simulink model "MPCquadprog"  (R2023a)
settings: Solver=ode4  StartTime=0.0  StopTime=tsim  FixedStep=baseRate  RelTol=1e-6  AbsTol=1e-6
values from neighbouring files (symbols this model uses):
  ALGORITHM = 5    [Run_Initializer.m]
  con0 = [n*N, 2*N, N, N, N]    [Run_Initializer.m]
  Gamma1_el = 0.12    [Run_Initializer.m]
  Gamma1_sh = 0.005    [Run_Initializer.m]
  Gamma1_wr = 0.025    [Run_Initializer.m]
  Gamma2_el = 5    [Run_Initializer.m]
  Gamma2_sh = 5    [Run_Initializer.m]
  Gamma2_wr = 5    [Run_Initializer.m]
  Gamma3_el = 10    [Run_Initializer.m]
  Gamma3_sh = 40    [Run_Initializer.m]
  Gamma3_wr = 40    [Run_Initializer.m]
  Gamma4_el = 0.039    [Run_Initializer.m]
  Gamma4_sh = 0.015    [Run_Initializer.m]
  Gamma4_wr = 0.029    [Run_Initializer.m]
  Gamma5_el = 800    [Run_Initializer.m]
  Gamma5_sh = 800    [Run_Initializer.m]
  Gamma5_wr = 800    [Run_Initializer.m]
  Gamma6_el = 0.000001    (= 1e-06)    [Run_Initializer.m]
  Gamma6_sh = 0.005    [Run_Initializer.m]
  Gamma6_wr = 0.02    [Run_Initializer.m]
  init_states_BLACK = [ct;thetat0].'    [Run_Initializer.m]
  init_states_BLUE = [pobj1;0].'    [Run_Initializer.m]
  init_states_RED = xi(1:3).'    [Run_Initializer.m]
  Kd_elarm = 0.8    [Run_Initializer.m]
  Kd_sharm = 1.0    (= 1)    [Run_Initializer.m]
  Kd_wrarm = 0.6    [Run_Initializer.m]
  Kp_elarm = 1.2    [Run_Initializer.m]
  Kp_sharm = 1.5    [Run_Initializer.m]
  Kp_wrarm = 2    [Run_Initializer.m]
  maxiterations = 10    [Run_Initializer.m]
  N = 15    [Run_Initializer.m]    (also in theConstraintLimits4.m)
  Td = 2    [Run_Initializer.m]
  thetat_dot = 2.5 * d2r    (= 0.0436332312999)    [Run_Initializer.m]
  tol = 0.00015    [Run_Initializer.m]
  Tz_lim_elarm = .1    (= 0.1)    [Run_Initializer.m]
  Tz_lim_sharm = .1    (= 0.1)    [Run_Initializer.m]
  Tz_lim_wrarm = .1    (= 0.1)    [Run_Initializer.m]
  vobj1 = [0.00;0.00]    [Run_Initializer.m]
  vtar = [-0.005;0.005]    [Run_Initializer.m]
undefined symbols (not defined in the file or in its folder): a1, a2, a3, Ad, b0, b1, b2, b3, baseRate, cdockdeltax, cdockoa, Cmat, DiscIntNeverNeededParam, drop_states_ARM, drop_states_BLACK, drop_states_BLUE, drop_states_RED, ecoa, F_Black_X_nominal, F_Black_Y_nominal, F_Blue_X_nominal, F_Blue_Y_nominal, F_red_X_nominal, F_red_Y_nominal, F_thrusters_BLACK, F_thrusters_BLUE, F_thrusters_RED, Fmat, gamma, H, IBLACK, IBLUE, IDIST, IEE, IPROX, IRED, Kd_tb, Kd_tblue, Kd_tr, Kd_xb, Kd_xblue, Kd_xr, Kd_yb, Kd_yblue, Kd_yr, KOZ_actual, Kp_tb, Kp_tblue, Kp_tr, Kp_xb, Kp_xblue, Kp_xr, Kp_yb, Kp_yblue, Kp_yr, mBLACK, mBLUE, mDIST, mEE, mPROX ... (+32)
libraries: nvidiaSharedBlocks x8, simulink x8, dspsigops x6, dspstat3 x5, MainLibrary x4
(part 10 of 10)

== matlab function MPCquadprog/Phase #3: Experiment/Change RED Behavior/Sub-Phase #4/Subsystem/MATLAB Function ==
  data: x input; x output
function x = fcn(x)
    if x > pi
        x  = x - 2*pi;
    elseif x <= -pi
        x = x + 2*pi;
    end

== matlab function MPCquadprog/Thruster Control Code/Change RED Behavior/Calculate Thruster ON//OFF/MATLAB Function3 ==
  data: H output; thruster_dist2CG_RED parameter; F_thrusters_RED parameter
function H = MakeH(thruster_dist2CG_RED,F_thrusters_RED)

Vec1 = [ -1
         -1
          0 
          0
          1
          1
          0
          0 ];
      
Vec2 = [  0
          0
          1
          1
          0
          0
         -1
         -1 ];
     
Vec3 = thruster_dist2CG_RED./1000;

Mat1 = [Vec1, Vec2, Vec3]';

Mat2 = diag((F_thrusters_RED./2));

H    = Mat1*Mat2;

end

== matlab function MPCquadprog/Thruster Control Code/Change RED Behavior/Calculate Thruster ON//OFF/MATLAB Function4 ==
  data: H output; thruster_dist2CG_RED parameter; F_red_X_nominal parameter; theta_1 input; theta_2 input; theta_3 input; mRED parameter; thrust_decay_factor input; F_red_Y_nominal parameter; mPROX parameter; mDIST parameter; mEE parameter; Phi parameter; b0 parameter; a1 parameter; b1 parameter; a2 parameter; b2 parameter; a3 parameter; b3 parameter
function H   = MakeH(thruster_dist2CG_RED,F_red_X_nominal, theta_1, theta_2, theta_3, mRED, thrust_decay_factor, F_red_Y_nominal, mPROX, mDIST, mEE, Phi, b0, a1, b1, a2, b2, a3, b3)
    
    link1_com_x = b0*cos(Phi) + a1*cos(pi/2 + theta_1);
    link1_com_y = b0*sin(Phi) + a1*sin(pi/2 + theta_1);
    
    link2_com_x = link1_com_x + b1*cos(pi/2 + theta_1) + a2*cos(pi/2 + theta_1 + theta_2);
    link2_com_y = link1_com_y + b1*sin(pi/2 + theta_1) + a2*sin(pi/2 + theta_1 + theta_2);
    
    link3_com_x = link2_com_x + b2*cos(pi/2 + theta_1 + theta_2) + a3*cos(pi/2 + theta_1 + theta_2 + theta_3);
    link3_com_y = link2_com_y + b2*sin(pi/2 + theta_1 + theta_2) + a3*sin(pi/2 + theta_1 + theta_2 + theta_3);
    
    delta_com_due_to_arm_x = (mPROX*link1_com_x + mDIST*link2_com_x + mEE*link3_com_x)/(mRED + mPROX + mDIST + mEE)*1000; % [mm]
    delta_com_due_to_arm_y = (mPROX*link1_com_y + mDIST*link2_com_y + mEE*link3_com_y)/(mRED + mPROX + mDIST + mEE)*1000; % [mm]
    
    adjusted_thruster_dist2CG_RED = [thruster_dist2CG_RED(1)-delta_com_due_to_arm_y;
                                     thruster_dist2CG_RED(2)-delta_com_due_to_arm_y;
                                     thruster_dist2CG_RED(3)-delta_com_due_to_arm_x;
                                     thruster_dist2CG_RED(4)-delta_com_due_to_arm_x;
                                     thruster_dist2CG_RED(5)+delta_com_due_to_arm_y;
                                     thruster_dist2CG_RED(6)+delta_com_due_to_arm_y;
                                     thruster_dist2CG_RED(7)+delta_com_due_to_arm_x;
                                     thruster_dist2CG_RED(8)+delta_com_due_to_arm_x];
                                     
    
    
    Vec1 = [ -1
             -1
              0 
              0
              1
              1
              0
              0 ];
          
    Vec2 = [  0
              0
              1
              1
              0
              0
             -1
             -1 ];
         
    Vec3 = adjusted_thruster_dist2CG_RED./1000;
    
    Mat1 = [Vec1, Vec2, Vec3]';
    
    F_thrusters_RED = [F_red_X_nominal*thrust_decay_factor; F_red_X_nominal*thrust_decay_factor; F_red_Y_nominal*thrust_decay_factor; F_red_Y_nominal*thrust_decay_factor; F_red_X_nominal*thrust_decay_factor; F_red_X_nominal*thrust_decay_factor; F_red_Y_nominal*thrust_decay_factor; F_red_Y_nominal*thrust_decay_factor];
    
    Mat2 = diag((F_thrusters_RED));
    
    H    = Mat1*Mat2;

end

== matlab function MPCquadprog/Thruster Control Code/Change RED Behavior/Calculate Thruster ON//OFF/MATLAB Function5 ==
  data: thrust_decay_factor output; PWMs input; thruster_count_threshold parameter; count output
function [thrust_decay_factor, count]  = check_thrust_decay(PWMs,thruster_count_threshold)

% normalize PWMs
if max(PWMs) > 1
    PWMs = PWMs/max(PWMs);
end

count = sum(PWMs > thruster_count_threshold);

positives_only = max(PWMs,0);
sum_of_duty_cycles = sum(positives_only);

average_duty_cycle_per_thruster = sum_of_duty_cycles/count;

% Look up the thrust decay for this average duty cycle
if (average_duty_cycle_per_thruster < 0.3) || (count == 0)
    thrust_decay_factor = 1;
else
    thrust_decay_factor = max(0.6 - 2*average_duty_cycle_per_thruster + 1, 0.5);   
end

== matlab function MPCquadprog/Thruster Control Code/Change RED Behavior/Calculate Thruster ON//OFF/MATLAB Function6 ==
  data: H output; thruster_dist2CG_RED parameter; F_red_X_nominal parameter; theta_1 input; theta_2 input; theta_3 input; mRED parameter; thrust_decay_factor input; F_red_Y_nominal parameter; mPROX parameter; mDIST parameter; mEE parameter; Phi parameter; b0 parameter; a1 parameter; b1 parameter; a2 parameter; b2 parameter; a3 parameter; b3 parameter
function H   = MakeHWithArmAndDecay(thruster_dist2CG_RED,F_red_X_nominal, theta_1, theta_2, theta_3,  mRED, thrust_decay_factor, F_red_Y_nominal, mPROX, mDIST, mEE, Phi, b0, a1, b1, a2, b2, a3, b3)
    
    link1_com_x = b0*cos(Phi) + a1*cos(pi/2 + theta_1);
    link1_com_y = b0*sin(Phi) + a1*sin(pi/2 + theta_1);
    
    link2_com_x = link1_com_x + b1*cos(pi/2 + theta_1) + a2*cos(pi/2 + theta_1 + theta_2);
    link2_com_y = link1_com_y + b1*sin(pi/2 + theta_1) + a2*sin(pi/2 + theta_1 + theta_2);
    
    link3_com_x = link2_com_x + b2*cos(pi/2 + theta_1 + theta_2) + a3*cos(pi/2 + theta_1 + theta_2 + theta_3);
    link3_com_y = link2_com_y + b2*sin(pi/2 + theta_1 + theta_2) + a3*sin(pi/2 + theta_1 + theta_2 + theta_3);
    
    delta_com_due_to_arm_x = (mPROX*link1_com_x + mDIST*link2_com_x + mEE*link3_com_x)/(mRED + mPROX + mDIST + mEE)*1000; % [mm]
    delta_com_due_to_arm_y = (mPROX*link1_com_y + mDIST*link2_com_y + mEE*link3_com_y)/(mRED + mPROX + mDIST + mEE)*1000; % [mm]
    
    adjusted_thruster_dist2CG_RED = [thruster_dist2CG_RED(1)-delta_com_due_to_arm_y;
                                     thruster_dist2CG_RED(2)-delta_com_due_to_arm_y;
                                     thruster_dist2CG_RED(3)-delta_com_due_to_arm_x;
                                     thruster_dist2CG_RED(4)-delta_com_due_to_arm_x;
                                     thruster_dist2CG_RED(5)+delta_com_due_to_arm_y;
                                     thruster_dist2CG_RED(6)+delta_com_due_to_arm_y;
                                     thruster_dist2CG_RED(7)+delta_com_due_to_arm_x;
                                     thruster_dist2CG_RED(8)+delta_com_due_to_arm_x];
                                 
    
    
    Vec1 = [ -1
             -1
              0 
              0
              1
              1
              0
              0 ];
          
    Vec2 = [  0
              0
              1
              1
              0
              0
             -1
             -1 ];
         
    Vec3 = adjusted_thruster_dist2CG_RED./1000;
    
    Mat1 = [Vec1, Vec2, Vec3]';
    
    F_thrusters_RED = [F_red_X_nominal*thrust_decay_factor; F_red_X_nominal*thrust_decay_factor; F_red_Y_nominal*thrust_decay_factor; F_red_Y_nominal*thrust_decay_factor; F_red_X_nominal*thrust_decay_factor; F_red_X_nominal*thrust_decay_factor; F_red_Y_nominal*thrust_decay_factor; F_red_Y_nominal*thrust_decay_factor];
    
    Mat2 = diag((F_thrusters_RED./2));
    
    H    = Mat1*Mat2;

end

== matlab function MPCquadprog/Phase #3: Experiment/Change RED Behavior/Sub-Phase #4/Subsystem/MATLAB Function2 ==
  data: x input; x output
function x = fcn(x)
    if x > pi
        x  = x - 2*pi;
    elseif x <= -pi
        x = x + 2*pi;
    end

== matlab function MPCquadprog/Phase #3: Experiment/Change BLACK Behavior/Sub-Phase #3 /Hough Control/MATLAB Function4 ==
  data: Oy input; e_out output; e_in input
function e_out = fcn(Oy, e_in)

a = sign(Oy'*e_in);
e_out = -a*norm(e_in);

== matlab function MPCquadprog/Phase #3: Experiment/Change BLACK Behavior/Sub-Phase #3 /Hough Control/MATLAB Function2 ==
  data: Oy output; z input; Ox output
function [Oy, Ox]   = C3( z )
%C3 gives the rotation matrix about the z-axis for an angle 'z'
%   z - the angle about the z-axis which you rotate
%   A - the rotation matrix

Ox = [cos(z) sin(z); -sin(z) cos(z)]*[1;0];
Oy = [cos(z) sin(z); -sin(z) cos(z)]*[0;1];
end

== matlab function MPCquadprog/Phase #3: Experiment/Change BLACK Behavior/Sub-Phase #3 /Hough Control/MATLAB Function3 ==
  data: z input; Ox output
function Ox    = C3( z )
%C3 gives the rotation matrix about the z-axis for an angle 'z'
%   z - the angle about the z-axis which you rotate
%   A - the rotation matrix

Ox = [cos(z) sin(z); -sin(z) cos(z)]*[1;0];
end

== matlab function MPCquadprog/Phase #3: Experiment/Change BLACK Behavior/Sub-Phase #1/Hough Control/MATLAB Function4 ==
  data: Oy input; e_out output; e_in input
function e_out = fcn(Oy, e_in)

a = sign(Oy'*e_in);
e_out = -a*norm(e_in);

== matlab function MPCquadprog/PhaseSpace Camera Code/Use Hardware to Obtain States/MATLAB Function ==
  data: StartClock output; RedReceiving input; BlackReceiving input; BlueReceiving input; platformSelection parameter
function StartClock = CheckForSync(RedReceiving, BlackReceiving, BlueReceiving, platformSelection)
        
    StartClock = 0;
    
    if (platformSelection == 1)
        
        if RedReceiving == 1

            StartClock = 1;

        else

            StartClock = 0;

        end
        
    elseif (platformSelection == 2)
        
        if BlackReceiving == 1

            StartClock = 1;

        else

            StartClock = 0;

        end  
        
    elseif (platformSelection == 3)
        
        if RedReceiving == 1 && BlackReceiving == 1

            StartClock = 1;

        else

            StartClock = 0;

        end    
        
    elseif (platformSelection == 4)
        
        if RedReceiving == 1 && BlackReceiving == 1

            StartClock = 1;

        else

            StartClock = 0;

        end
        
    elseif (platformSelection == 5)
        
        if RedReceiving == 1

            StartClock = 1;

        else

            StartClock = 0;

        end
        
    elseif (platformSelection == 6)
        
        if BlueReceiving == 1

            StartClock = 1;

        else

            StartClock = 0;

        end
        
    elseif (platformSelection == 7)
        
        if RedReceiving == 1 && BlueReceiving == 1

            StartClock = 1;

        else

            StartClock = 0;

        end
        
    elseif (platformSelection == 8)
        
        if RedReceiving == 1 && BlackReceiving == 1 && BlueReceiving == 1

            StartClock = 1;

        else

            StartClock = 0;

        end
        
    elseif (platformSelection == 9)
        
        if BlackReceiving == 1 && BlueReceiving == 1

            StartClock = 1;

        else

            StartClock = 0;

        end
                           
    elseif (platformSelection == 10)
        
        if RedReceiving == 1 && BlueReceiving == 1

            StartClock = 1;

        else

            StartClock = 0;

        end
        
    elseif (platformSelection == 11)
        
        if RedReceiving == 1 && BlackReceiving == 1 && BlueReceiving == 1

            StartClock = 1;

        else

            StartClock = 0;

        end
        
    end



end

== matlab function MPCquadprog/Thruster Control Code/Change BLUE Behavior/Calculate Thruster ON//OFF/MATLAB Function6 ==
  data: thrust_decay_factor output; PWMs input; thruster_count_threshold parameter; count output
function [thrust_decay_factor, count]  = check_thrust_decay(PWMs,thruster_count_threshold)

% normalize PWMs
if max(PWMs) > 1
    PWMs = PWMs/max(PWMs);
end

count = sum(PWMs > thruster_count_threshold);

positives_only = max(PWMs,0);
sum_of_duty_cycles = sum(positives_only);

average_duty_cycle_per_thruster = sum_of_duty_cycles/count;

% Look up the thrust decay for this average duty cycle
if (average_duty_cycle_per_thruster < 0.3) || (count == 0)
    thrust_decay_factor = 1;
else
    thrust_decay_factor = max(0.6 - 2*average_duty_cycle_per_thruster + 1, 0.5);   
end

== matlab function MPCquadprog/Thruster Control Code/Change BLUE Behavior/Calculate Thruster ON//OFF/MATLAB Function7 ==
  data: H output; thruster_dist2CG_BLUE parameter; F_Blue_X_nominal parameter; thrust_decay_factor input; F_Blue_Y_nominal parameter
function H   = MakeHWithDecay(thruster_dist2CG_BLUE,F_Blue_X_nominal, thrust_decay_factor, F_Blue_Y_nominal)


adjusted_thruster_dist2CG_BLUE = [thruster_dist2CG_BLUE(1);
                                 thruster_dist2CG_BLUE(2);
                                 thruster_dist2CG_BLUE(3);
                                 thruster_dist2CG_BLUE(4);
                                 thruster_dist2CG_BLUE(5);
                                 thruster_dist2CG_BLUE(6);
                                 thruster_dist2CG_BLUE(7);
                                 thruster_dist2CG_BLUE(8)];
                                 


Vec1 = [ -1
         -1
          0 
          0
          1
          1
          0
          0 ];
      
Vec2 = [  0
          0
          1
          1
          0
          0
         -1
         -1 ];
     
Vec3 = adjusted_thruster_dist2CG_BLUE./1000;

Mat1 = [Vec1, Vec2, Vec3]';

F_thrusters_BLUE = [F_Blue_X_nominal*thrust_decay_factor; F_Blue_X_nominal*thrust_decay_factor; F_Blue_Y_nominal*thrust_decay_factor; F_Blue_Y_nominal*thrust_decay_factor; F_Blue_X_nominal*thrust_decay_factor; F_Blue_X_nominal*thrust_decay_factor; F_Blue_Y_nominal*thrust_decay_factor; F_Blue_Y_nominal*thrust_decay_factor];

Mat2 = diag((F_thrusters_BLUE./2));

H    = Mat1*Mat2;

end

== matlab function MPCquadprog/Phase #3: Experiment/Change BLUE Behavior/Sub-Phase #2 /Hough Control/MATLAB Function2 ==
  data: Oy output; z input; Ox output
function [Oy, Ox]   = C3( z )
%C3 gives the rotation matrix about the z-axis for an angle 'z'
%   z - the angle about the z-axis which you rotate
%   A - the rotation matrix

Ox = [cos(z) sin(z); -sin(z) cos(z)]*[1;0];
Oy = [cos(z) sin(z); -sin(z) cos(z)]*[0;1];
end

== matlab function MPCquadprog/Thruster Control Code/Change BLACK Behavior/Calculate Thruster ON//OFF/MATLAB Function10 ==
  data: thrust_decay_factor output; PWMs input; thruster_count_threshold parameter; count output
function [thrust_decay_factor, count]  = check_thrust_decay(PWMs,thruster_count_threshold)

% normalize PWMs
if max(PWMs) > 1
    PWMs = PWMs/max(PWMs);
end

count = sum(PWMs > thruster_count_threshold);

positives_only = max(PWMs,0);
sum_of_duty_cycles = sum(positives_only);

average_duty_cycle_per_thruster = sum_of_duty_cycles/count;

% Look up the thrust decay for this average duty cycle
if (average_duty_cycle_per_thruster < 0.3) || (count == 0)
    thrust_decay_factor = 1;
else
    thrust_decay_factor = max(0.6 - 2*average_duty_cycle_per_thruster + 1, 0.5);   
end

== matlab function MPCquadprog/Thruster Control Code/Change BLACK Behavior/Calculate Thruster ON//OFF/MATLAB Function11 ==
  data: H output; thruster_dist2CG_BLACK parameter; F_Black_X_nominal parameter; thrust_decay_factor input; F_Black_Y_nominal parameter
function H   = MakeHWithDecay(thruster_dist2CG_BLACK,F_Black_X_nominal, thrust_decay_factor, F_Black_Y_nominal)


adjusted_thruster_dist2CG_BLACK = [thruster_dist2CG_BLACK(1);
                                 thruster_dist2CG_BLACK(2);
                                 thruster_dist2CG_BLACK(3);
                                 thruster_dist2CG_BLACK(4);
                                 thruster_dist2CG_BLACK(5);
                                 thruster_dist2CG_BLACK(6);
                                 thruster_dist2CG_BLACK(7);
                                 thruster_dist2CG_BLACK(8)];
                                 


Vec1 = [ -1
         -1
          0 
          0
          1
          1
          0
          0 ];
      
Vec2 = [  0
          0
          1
          1
          0
          0
         -1
         -1 ];
     
Vec3 = adjusted_thruster_dist2CG_BLACK./1000;

Mat1 = [Vec1, Vec2, Vec3]';

F_thrusters_BLACK = [F_Black_X_nominal*thrust_decay_factor; F_Black_X_nominal*thrust_decay_factor; F_Black_Y_nominal*thrust_decay_factor; F_Black_Y_nominal*thrust_decay_factor; F_Black_X_nominal*thrust_decay_factor; F_Black_X_nominal*thrust_decay_factor; F_Black_Y_nominal*thrust_decay_factor; F_Black_Y_nominal*thrust_decay_factor];

Mat2 = diag((F_thrusters_BLACK./2));

H    = Mat1*Mat2;

end

== matlab function MPCquadprog/Phase #3: Experiment/Change BLUE Behavior/Sub-Phase #3 /Hough Control/MATLAB Function2 ==
  data: Oy output; z input; Ox output
function [Oy, Ox]   = C3( z )
%C3 gives the rotation matrix about the z-axis for an angle 'z'
%   z - the angle about the z-axis which you rotate
%   A - the rotation matrix

Ox = [cos(z) sin(z); -sin(z) cos(z)]*[1;0];
Oy = [cos(z) sin(z); -sin(z) cos(z)]*[0;1];
end

== matlab function MPCquadprog/Phase #3: Experiment/Change BLUE Behavior/Sub-Phase #3 /Hough Control/MATLAB Function3 ==
  data: z input; Ox output
function Ox    = C3( z )
%C3 gives the rotation matrix about the z-axis for an angle 'z'
%   z - the angle about the z-axis which you rotate
%   A - the rotation matrix

Ox = [cos(z) sin(z); -sin(z) cos(z)]*[1;0];
end

== matlab function MPCquadprog/Phase #3: Experiment/Change BLUE Behavior/Sub-Phase #3 /Hough Control/MATLAB Function4 ==
  data: Oy input; e_out output; e_in input
function e_out = fcn(Oy, e_in)

a = sign(Oy'*e_in);
e_out = -a*norm(e_in);

== matlab function MPCquadprog/Phase #3: Experiment/Change BLUE Behavior/Sub-Phase #2 /Hough Control/MATLAB Function3 ==
  data: z input; Ox output
function Ox    = C3( z )
%C3 gives the rotation matrix about the z-axis for an angle 'z'
%   z - the angle about the z-axis which you rotate
%   A - the rotation matrix

Ox = [cos(z) sin(z); -sin(z) cos(z)]*[1;0];
end

== matlab function MPCquadprog/Phase #3: Experiment/Change BLUE Behavior/Sub-Phase #4/Hough Control/MATLAB Function2 ==
  data: Oy output; z input; Ox output
function [Oy, Ox]   = C3( z )
%C3 gives the rotation matrix about the z-axis for an angle 'z'
%   z - the angle about the z-axis which you rotate
%   A - the rotation matrix

Ox = [cos(z) sin(z); -sin(z) cos(z)]*[1;0];
Oy = [cos(z) sin(z); -sin(z) cos(z)]*[0;1];
end

== matlab function MPCquadprog/Phase #3: Experiment/Change BLUE Behavior/Sub-Phase #4/Hough Control/MATLAB Function3 ==
  data: z input; Ox output
function Ox    = C3( z )
%C3 gives the rotation matrix about the z-axis for an angle 'z'
%   z - the angle about the z-axis which you rotate
%   A - the rotation matrix

Ox = [cos(z) sin(z); -sin(z) cos(z)]*[1;0];
end
